simulink model "Dice_HW_start_2025"  (R2024b)
settings: Solver=FixedStepAuto  StartTime=0.0  StopTime=inf  RelTol=1e-3
libraries: microbitledlib x8, microbitaccellib x2
settings Model: SimulationMode=external  ExtModeTrigDuration=5  Creator=The MathWorks, Inc.  LastModifiedBy=ahenshaw
settings SolverCC: AlgebraicLoopSolver=TrustRegion
settings DataIOCC: ReturnWorkspaceOutputs=off
settings OptimizationCC: MaxStackSize=64
settings DebuggingCC: ParameterTunabilityLossMsg=error  UnconnectedInputMsg=warning  UnconnectedOutputMsg=warning  UnconnectedLineMsg=warning  ArithmeticOperatorsInVariantConditions=warning
settings HardwareCC: ProdBitPerPointer=32  ProdBitPerSizeT=32  ProdBitPerPtrDiffT=32  ProdLargestAtomicInteger=Long  ProdLargestAtomicFloat=Double  ProdWordSize=32  ProdHWDeviceType=ARM Compatible->ARM Cortex
settings ModelReferenceCC: EnableRefExpFcnMdlSchedulingChecks=on
settings SFSimCC: SimUseLocalCustomCode=off  CustomCodeUndefinedFunction=UseInterfaceOnly
settings RTWCC: Description=Embedded Coder  SystemTargetFile=ert.tlc  HardwareBoard=BBC micro:bit V2  TemplateMakefile=ert_default_tmf  RTWUseLocalCustomCode=off  Toolchain=GNU Tools for ARM Embedded Processors  GPUComputeCapability=3.5
settings CodeAppCC: ForceParamTrailComments=on  OperatorAnnotations=on  StateflowObjectComments=on  MATLABSourceComments=on
settings ERTTargetCC: MultiwordLength=2048  ERTCustomFileBanners=off  SupportContinuousTime=on  SupportNonInlinedSFcns=on  RemoveResetFunc=off  ModelStepFunctionPrototypeControlCompliant=off  ExtModeTransport=3  ExtModeStaticAlloc=on  ExtModeMexFile=ext_xcp  ExtModeIntrfLevel=Level2 - Open  InlinedParameterPlacement=Hierarchical  DynamicArrayContainerType=coder::array

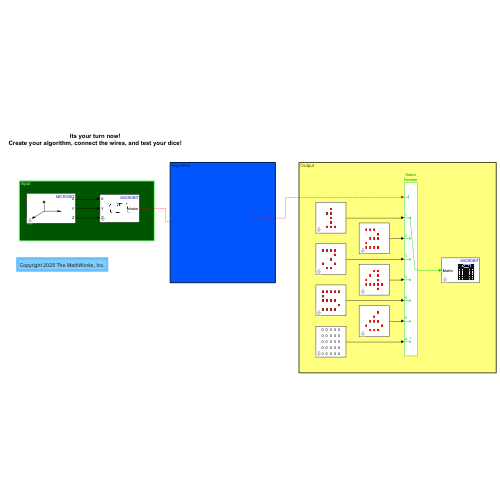
[thumbnail: Simulink's stored preview of the top-level diagram]
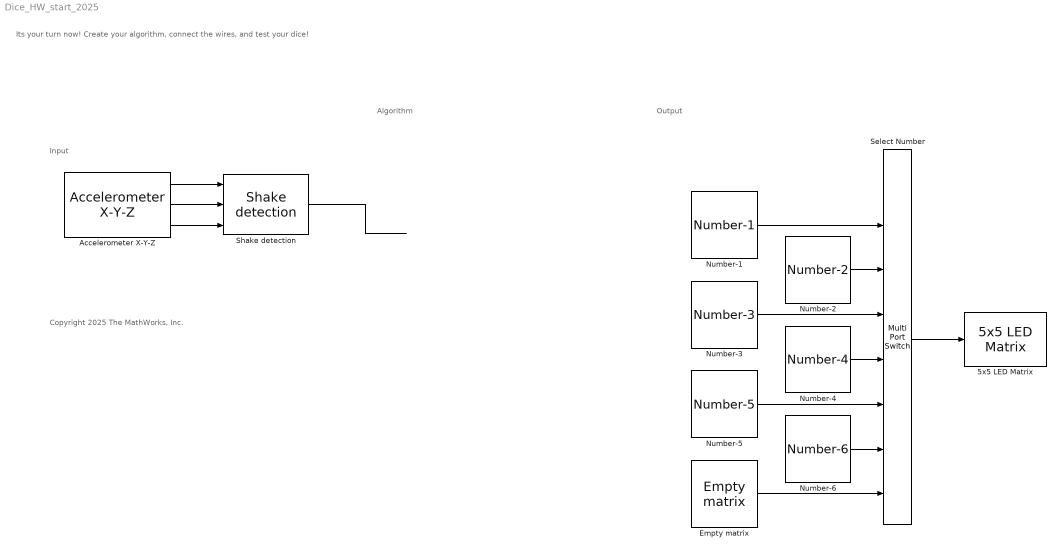
== system Dice_HW_start_2025 ==
  note: Its your turn now!
      | Create your algorithm, connect the wires, and test your dice!
  note: Input
  note: Output
  note: Algorithm
  note: Copyright 2025 The MathWorks, Inc.
  5x5 LED Matrix : microbitledlib/5x5 LED Matrix  LED_mat=[0 1 1 1 0;1 0 1 0 1;1 1 0 1 1; 1 0 1 0 1;0 1 1 1 0]
  Accelerometer X-Y-Z : microbitaccellib/Accelerometer X-Y-Z  ODR=800Hz  Accelfullrange=-2g to +2g  SampleTime=0.1
  Empty matrix : microbitledlib/LED Images/Empty matrix  L00=off  L01=off  L02=off  L03=off  L04=off  L10=off  L11=off  L12=off  L13=off  L14=off  L20=off  L21=off  L22=off  L23=off  L24=off  L30=off  L31=off  L32=off  L33=off  L34=off  L40=off  L41=off  L42=off  L43=off  L44=off
  Number-1 : microbitledlib/LED Images/Number-1  L00=off  L01=off  L02=on  L03=off  L04=off  L10=off  L11=on  L12=on  L13=off  L14=off  L20=off  L21=off  L22=on  L23=off  L24=off  L30=off  L31=off  L32=on  L33=off  L34=off  L40=off  L41=on  L42=on  L43=on  L44=off
  Number-2 : microbitledlib/LED Images/Number-2  L00=on  L01=on  L02=on  L03=off  L04=off  L10=off  L11=off  L12=off  L13=on  L14=off  L20=off  L21=on  L22=on  L23=on  L24=off  L30=on  L31=off  L32=off  L33=off  L34=off  L40=on  L41=on  L42=on  L43=on  L44=off
  Number-3 : microbitledlib/LED Images/Number-3  L00=on  L01=on  L02=on  L03=on  L04=off  L10=off  L11=off  L12=off  L13=on  L14=off  L20=off  L21=off  L22=on  L23=off  L24=off  L30=on  L31=off  L32=off  L33=on  L34=off  L40=off  L41=on  L42=on  L43=off  L44=off
  Number-4 : microbitledlib/LED Images/Number-4  L00=off  L01=off  L02=on  L03=on  L04=off  L10=off  L11=on  L12=off  L13=on  L14=off  L20=on  L21=off  L22=off  L23=on  L24=off  L30=on  L31=on  L32=on  L33=on  L34=on  L40=off  L41=off  L42=off  L43=on  L44=off
  Number-5 : microbitledlib/LED Images/Number-5  L00=on  L01=on  L02=on  L03=on  L04=on  L10=on  L11=off  L12=off  L13=off  L14=off  L20=on  L21=on  L22=on  L23=on  L24=off  L30=off  L31=off  L32=off  L33=off  L34=on  L40=on  L41=on  L42=on  L43=on  L44=off
  Number-6 : microbitledlib/LED Images/Number-6  L00=off  L01=off  L02=off  L03=on  L04=off  L10=off  L11=off  L12=on  L13=off  L14=off  L20=off  L21=on  L22=on  L23=on  L24=off  L30=on  L31=off  L32=off  L33=off  L34=on  L40=off  L41=on  L42=on  L43=on  L44=off
  Select Number : MultiPortSwitch  Inputs=7  DiagnosticForDefault=None  SaturateOnIntegerOverflow=off  InputSameDT=off
  Shake detection : microbitaccellib/Shake detection  sen=2
  wires:
  Accelerometer X-Y-Z/1 -> Shake detection/1
  Accelerometer X-Y-Z/2 -> Shake detection/2
  Accelerometer X-Y-Z/3 -> Shake detection/3
  Number-1/1 -> Select Number/2
  Number-2/1 -> Select Number/3
  Number-3/1 -> Select Number/4
  Number-4/1 -> Select Number/5
  Number-5/1 -> Select Number/6
  Number-6/1 -> Select Number/7
  Empty matrix/1 -> Select Number/8
  Select Number/1 -> 5x5 LED Matrix/1
  ? -> Select Number/1
  Shake detection/1 -> ?
